simulink model "Simulation_Assignment_4_2015297"  (R2016a)
settings: Solver=VariableStepAuto  StartTime=0.0  StopTime=100  RelTol=1e-3
settings Model: Creator=hp  LastModifiedBy=hp

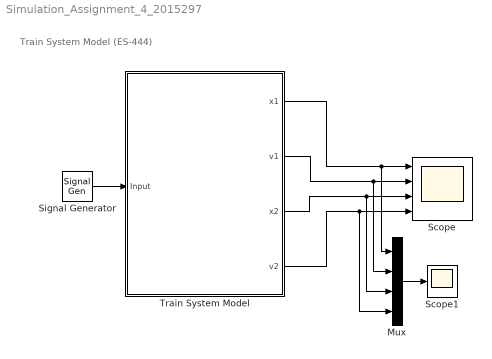
== system Simulation_Assignment_4_2015297 ==
  note: Train System Model (ES-444)
  Mux : Mux
  Scope : Scope  NumInputPorts=4
  Scope1 : Scope
  Signal Generator : SignalGenerator  WaveForm=square  Amplitude=-1  Frequency=0.001  Units=rad/sec
  Train System Model : Subsystem  mask{M1=1, M2=0.5, k=40, mu=0.0002, g=9.8}
      mask prompts: M1 "Mass of Engine (kg)"; M2 "Mass of Car (kg)"; k "Spring Constant (N/sec)"; mu "Coefficient of Rolling Friction (sec/m)"; g "Gravity (m/sec^2)"
  wires:
  Train System Model/1(x1) -> Mux/1, Scope/1
  Train System Model/2(v1) -> Mux/2, Scope/2
  Train System Model/3(x2) -> Mux/3, Scope/3
  Train System Model/4(v2) -> Mux/4, Scope/4
  Mux/1 -> Scope1/1
  Signal Generator/1 -> Train System Model/1(Input)

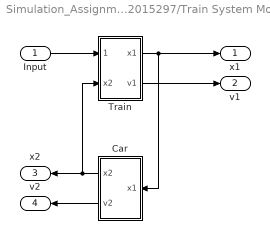
== system Simulation_Assignment_4_2015297/Train System Model ==
  Input : Inport
  Car : Subsystem
  Train : Subsystem
  x1 : Outport
  v1 : Outport  Port=2
  x2 : Outport  Port=3
  v2 : Outport  Port=4
  wires:
  Input/1 -> Train/1(Input)
  Train/1(x1) -> Car/1(x1), x1/1
  Car/1(x2) -> x2/1, Train/2(x2)
  Train/2(v1) -> v1/1
  Car/2(v2) -> v2/1

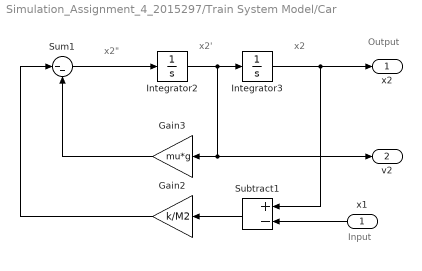
== system Simulation_Assignment_4_2015297/Train System Model/Car ==
  note: Output
  note: x2"
  note: x2'
  note: x2
  note: Input
  x1 : Inport
  Gain2 : Gain  Gain=k/M2
  Gain3 : Gain  Gain=mu*g
  Integrator2 : Integrator
  Integrator3 : Integrator
  Subtract1 : Sum  Inputs=+-
  Sum1 : Sum  Inputs=|--
  x2 : Outport
  v2 : Outport  Port=2
  wires:
  x1/1 -> Subtract1/2
  Sum1/1 -> Integrator2/1
  Integrator2/1 -> v2/1, Gain3/1, Integrator3/1
  Gain2/1 -> Sum1/1
  Gain3/1 -> Sum1/2
  Subtract1/1 -> Gain2/1
  Integrator3/1 -> x2/1, Subtract1/1

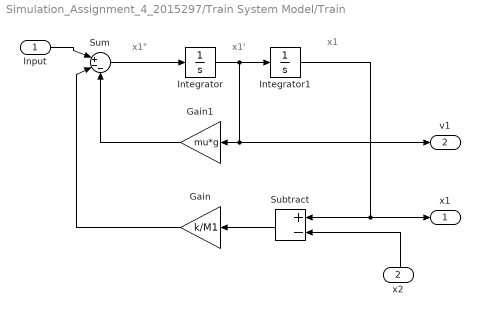
== system Simulation_Assignment_4_2015297/Train System Model/Train ==
  note: x1"
  note: x1'
  note: x1
  Input : Inport
  x2 : Inport  Port=2
  Gain : Gain  Gain=k/M1
  Gain1 : Gain  Gain=mu*g
  Integrator : Integrator
  Integrator1 : Integrator
  Subtract : Sum  Inputs=+-
  Sum : Sum  Inputs=|+--
  x1 : Outport
  v1 : Outport  Port=2
  wires:
  x2/1 -> Subtract/2
  Subtract/1 -> Gain/1
  Gain1/1 -> Sum/3
  Gain/1 -> Sum/2
  Input/1 -> Sum/1
  Integrator1/1 -> x1/1, Subtract/1
  Sum/1 -> Integrator/1
  Integrator/1 -> Gain1/1, v1/1, Integrator1/1
